simulink library "libAggregators"  (R2015a)
settings: Solver=ode45  StartTime=0.0  StopTime=10.0  RelTol=1e-3
libraries: dspsigattribs x4, libAggregators x1
settings Model: Creator=jcardena  LastModifiedBy=jcardena
settings DebuggingCC: UnderspecifiedInitializationDetection=Classic  MergeDetectMultiDrivingBlocksExec=none  SolverPrmCheckMsg=warning  StateNameClashWarn=warning

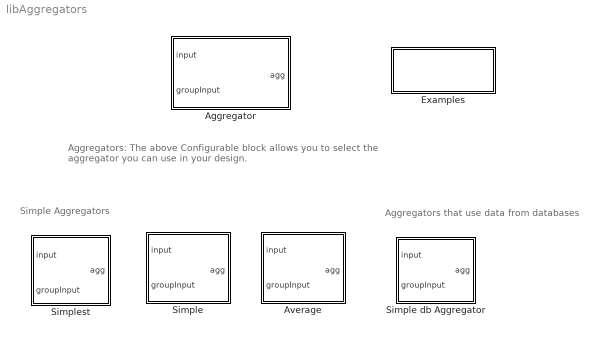
== system libAggregators ==
  note: Aggregators that use data from databases
  note: Simple Aggregators
  note: Aggregators: The above Configurable block allows you to select the aggregator you can use in your design.
  Aggregator : Subsystem  BlockChoice=Average
      settings: TemplateBlock=self  MemberBlocks=Average,Simple,Simple db Aggregator,Simplest
  Average : Subsystem  mask(aggregatingBlock){gVal=1}
      mask prompts: gVal "Grouping expression or value"
      mask help: An Aggregator classifies data rows from a single input link into groups and computes totals or other aggregate functions for each group. The averaged totals for each group are output from the stage via an output port.
      settings: RTWFcnNameOpts=Use subsystem name  RTWFileNameOpts=Use function name
      mask Help: Enter the aggregate function
      mask Display: image('images/aggrIcon.png')
  Examples : Subsystem  mask(Aggregator Examples){}
      mask Display: disp('Aggregator\nExamples')
  Simple : Subsystem  mask(aggregatingBlock){gVal=1}
      mask prompts: gVal "Grouping expression or value"
      mask help: An Aggregator classifies data rows from a single input link into groups and computes totals or other aggregate functions for each group. The summed totals for each group are output from the stage via an output port.
      mask Help: Enter the aggregate function
      mask Display: image('images/aggrIcon.png')
  Simple db Aggregator : Subsystem
      mask Display: image('images/aggrIcon.png')
  Simplest : Subsystem
      mask Display: image('images/aggrIcon.png')

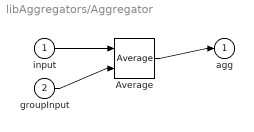
== system libAggregators/Aggregator ==
  input : Inport
  groupInput : Inport  Port=2
  Average : libAggregators/Average  gVal=1
  agg : Outport
  wires:
  input/1 -> Average/1
  groupInput/1 -> Average/2
  Average/1 -> agg/1

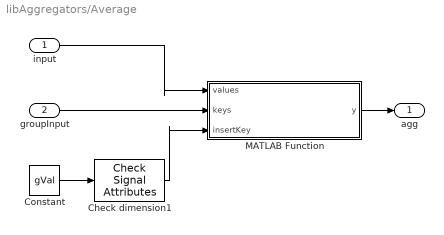
== system libAggregators/Average ==
  input : Inport
  groupInput : Inport  Port=2
  Check dimension1 : dspsigattribs/Check Signal Attributes  SigAttribCheckMethod=Does not match attributes exactly  Complexity=Ignore  Frame=Ignore  DimsCheckMethod=Is...  Dimensions=Vector (1-D or 2-D)  DatatypeCheckMethod=Ignore  DatatypeGeneral=Floating-point  DtypeFloatSpecific=Any floating-point  DtypeFixedSpecific=Any fixed-point  DtypeIntSpecific=Any integer  SampleMode=Ignore
  Constant : Constant  Value=gVal
  MATLAB Function : MATLAB Function  TreatAsAtomicUnit=on
      settings: RTWSystemCode=Inline
  agg : Outport
  wires:
  input/1 -> MATLAB Function/1(values)
  groupInput/1 -> MATLAB Function/2(keys)
  Constant/1 -> Check dimension1/1
  MATLAB Function/1(y) -> agg/1
  Check dimension1/1 -> MATLAB Function/3(insertKey)

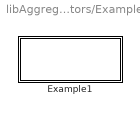
== system libAggregators/Examples ==
  Example1 : Subsystem
      settings: OpenFcn=read_simulated_unitIDs_example

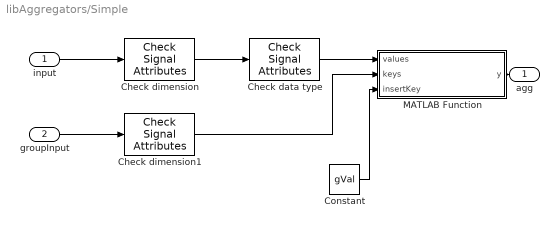
== system libAggregators/Simple ==
  input : Inport
  groupInput : Inport  Port=2
  Check data type : dspsigattribs/Check Signal Attributes  SigAttribCheckMethod=Does not match attributes exactly  Complexity=Ignore  Frame=Ignore  DimsCheckMethod=Ignore  Dimensions=Full matrix (2-D)  DatatypeCheckMethod=Is...  DatatypeGeneral=Floating-point  DtypeFloatSpecific=Double precision  DtypeFixedSpecific=Any fixed-point  DtypeIntSpecific=Any integer  SampleMode=Ignore
  Check dimension : dspsigattribs/Check Signal Attributes  SigAttribCheckMethod=Does not match attributes exactly  Complexity=Ignore  Frame=Ignore  DimsCheckMethod=Is...  Dimensions=Vector (1-D or 2-D)  DatatypeCheckMethod=Ignore  DatatypeGeneral=Floating-point  DtypeFloatSpecific=Any floating-point  DtypeFixedSpecific=Any fixed-point  DtypeIntSpecific=Any integer  SampleMode=Ignore
  Check dimension1 : dspsigattribs/Check Signal Attributes  SigAttribCheckMethod=Does not match attributes exactly  Complexity=Ignore  Frame=Ignore  DimsCheckMethod=Is...  Dimensions=Vector (1-D or 2-D)  DatatypeCheckMethod=Ignore  DatatypeGeneral=Floating-point  DtypeFloatSpecific=Any floating-point  DtypeFixedSpecific=Any fixed-point  DtypeIntSpecific=Any integer  SampleMode=Ignore
  Constant : Constant  Value=gVal
  MATLAB Function : MATLAB Function  TreatAsAtomicUnit=on
      settings: RTWSystemCode=Inline
  agg : Outport
  wires:
  groupInput/1 -> Check dimension1/1
  Check dimension/1 -> Check data type/1
  input/1 -> Check dimension/1
  Check dimension1/1 -> MATLAB Function/2(keys)
  MATLAB Function/1(y) -> agg/1
  Check data type/1 -> MATLAB Function/1(values)
  Constant/1 -> MATLAB Function/3(insertKey)

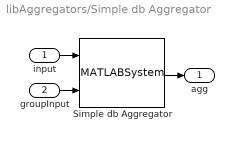
== system libAggregators/Simple db Aggregator ==
  input : Inport
  groupInput : Inport  Port=2
  Simple db Aggregator : MATLABSystem  System=db_Aggregator_mtlbSysBlock  SimulateUsing=Code generation
      mask Type: db_Aggregator_mtlbSysBlock
      mask Display:
      | disp('db_Aggregator_mtlbSysBlock');
      | port_label('input',1,'input');
      | port_label('input',2,'gropuInput');
      | port_label('output',1,'agg');
  agg : Outport
  wires:
  input/1 -> Simple db Aggregator/1
  groupInput/1 -> Simple db Aggregator/2
  Simple db Aggregator/1 -> agg/1

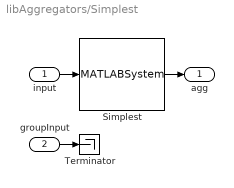
== system libAggregators/Simplest ==
  input : Inport
  groupInput : Inport  Port=2
  Simplest : MATLABSystem  System=simplestAggregator_mtlbSysBlock
      mask Type: simplestAggregator_mtlbSysBlock
      mask Display:
      | disp('Simplest');
      | port_label('input',1,'u');
      | port_label('output',1,'agg');
  Terminator : Terminator
  agg : Outport
  wires:
  input/1 -> Simplest/1
  Simplest/1 -> agg/1
  groupInput/1 -> Terminator/1

== system libAggregators/Examples/Example1 ==

== matlab function libAggregators/Average/MATLAB Function ==
  data: values input; y output; keys input; insertKey input
function y = avgAggr(values, keys, insertKey)
%#codegen
index = keys == insertKey;
y = mean(values(index));

== matlab function libAggregators/Simple/MATLAB Function ==
  data: values input; y output; keys input; insertKey input
function y = sumAggr(values, keys, insertKey)
%#codegen
index = keys == insertKey;
y = sum(values(index));
